simulink model "Exercise19real"  (Simulink 7.2)
settings: Solver=ode45  StartTime=0.0  StopTime=10.0  RelTol=1e-3
libraries: simulink x1
settings Model: Creator=Inderjot  LastModifiedBy=Inderjot

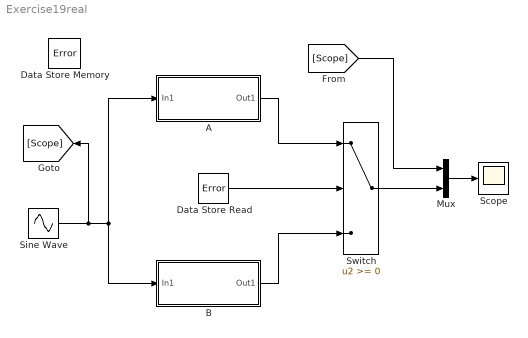
== system Exercise19real ==
  A : Subsystem
  B : Subsystem
  Data Store Memory : DataStoreMemory  DataStoreName=Error  ReadBeforeWriteMsg=warning  WriteAfterWriteMsg=warning  WriteAfterReadMsg=warning  OutDataType=sfix(16)  OutScaling=2^0
  Data Store Read : DataStoreRead  DataStoreName=Error  SampleTime=0
  Mux : Mux  Inputs=2
  Scope : Scope
  Sine Wave : Sin  SampleTime=0.1
  Switch : Switch  OutDataType=sfix(16)  OutScaling=2^0
  wires:
  Sine Wave/1 -> A/1(In1), B/1(In1), [Scope]
  A/1(Out1) -> Switch/1
  Data Store Read/1 -> Switch/2
  B/1(Out1) -> Switch/3
  Switch/1 -> Mux/2
  [Scope] -> Mux/1
  Mux/1 -> Scope/1

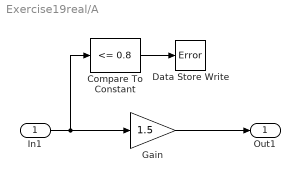
== system Exercise19real/A ==
  In1 : Inport  OutDataType=sfix(16)  OutScaling=2^0
  Compare To Constant : simulink/Logic and Bit Operations/Compare To Constant  SystemSampleTime=-1  relop=<=  const=0.8  LogicOutDataTypeMode=boolean  ZeroCross=off
  Data Store Write : DataStoreWrite  DataStoreName=Error  SampleTime=-1
  Gain : Gain  Gain=1.5  ParameterDataType=sfix(16)  ParameterScaling=2^0  OutDataType=sfix(16)  OutScaling=2^0
  Out1 : Outport  OutDataType=sfix(16)  OutScaling=2^0
  wires:
  Compare To Constant/1 -> Data Store Write/1
  In1/1 -> Gain/1, Compare To Constant/1
  Gain/1 -> Out1/1

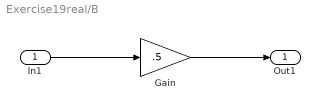
== system Exercise19real/B ==
  In1 : Inport  OutDataType=sfix(16)  OutScaling=2^0
  Gain : Gain  Gain=.5  ParameterDataType=sfix(16)  ParameterScaling=2^0  OutDataType=sfix(16)  OutScaling=2^0
  Out1 : Outport  OutDataType=sfix(16)  OutScaling=2^0
  wires:
  In1/1 -> Gain/1
  Gain/1 -> Out1/1
